simulink model "DCDC1_CL"  (R2024a)
settings: Solver=VariableStepAuto  StartTime=0.0  StopTime=Tsim_outLoop  FixedStep=Tstep  RelTol=1e-3
undefined symbols (not defined in the file): deadtimesw, den_aaf, DiscIntNeverNeededParam, ILmax, kaw_i, kaw_v, ki_i, ki_v, kp_i, kp_v, kpf_i, kpf_v, num_aaf, Rload, Tstep, Tsw, VinNom, VLlim, VoutNom, zden_pf_i, zden_pf_v, znum_pf_i, znum_pf_v
libraries: nesl_utility x12, fl_lib x11, simulink x6, ee_lib x3, spsTriangleGeneratorLib x2
settings Model: Creator=nicholas  LastModifiedBy=nicholas
settings RTWCC: GPUComputeCapability=3.5

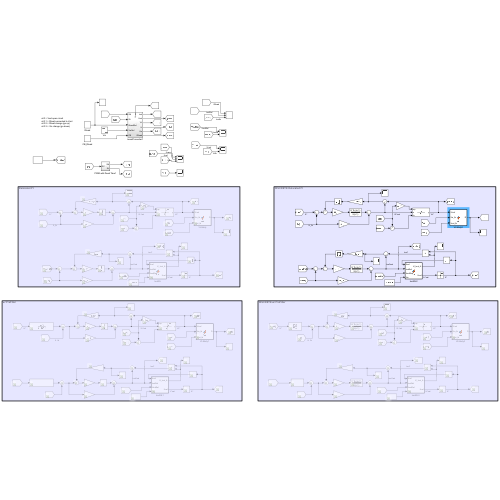
[thumbnail: Simulink's stored preview of the top-level diagram]
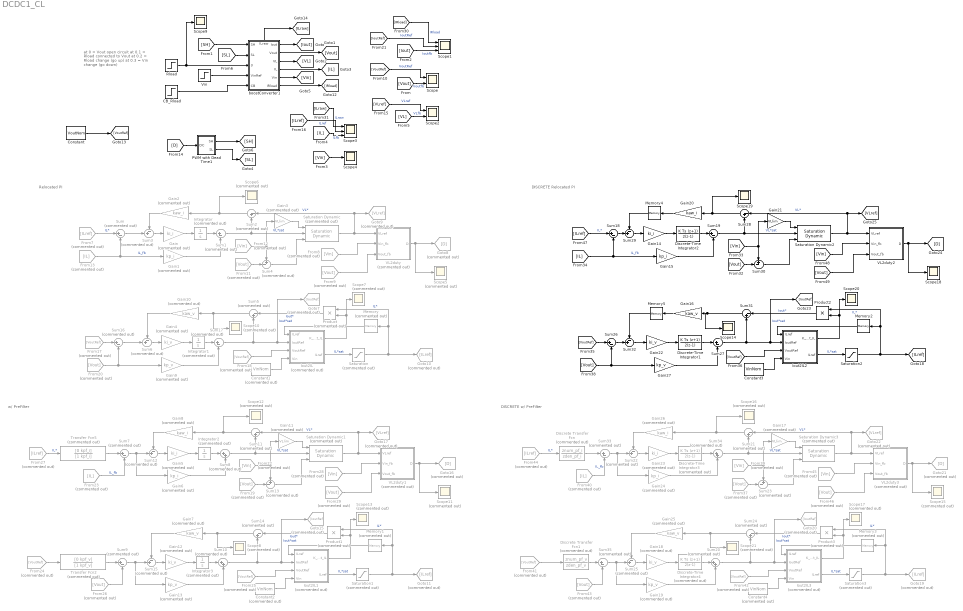
== system DCDC1_CL ==
  note: at 0 = Vout open circuit
      | at 0.1 = Rload connected to Vout
      | at 0.2 = Rload change (go up)
      | at 0.3 = Vin change (go down)
  note: Relocated PI
  note: w/ PreFilter
  note: DISCRETE w/ PreFilter
  note: DISCRETE Relocated PI
  CB_Rload : Step  Time=0.1  SampleTime=0
  Constant : Constant  Value=VoutNom
  Constant1 : Constant  Commented=on  Value=VinNom
  Constant2 : Constant  Commented=on  Value=VinNom
  Constant3 : Constant  Value=VinNom
  Constant4 : Constant  Commented=on  Value=VinNom
  Discrete Transfer Fcn : DiscreteTransferFcn  Commented=on  Numerator=znum_pf_i  Denominator=zden_pf_i
  Discrete Transfer Fcn1 : DiscreteTransferFcn  Commented=on  Numerator=znum_pf_v  Denominator=zden_pf_v
  Discrete-Time Integrator1 : DiscreteIntegrator  IntegratorMethod=Integration: Trapezoidal  SampleTime=Tsw  ICPrevOutput=DiscIntNeverNeededParam  ICPrevScaledInput=DiscIntNeverNeededParam
  Discrete-Time Integrator2 : DiscreteIntegrator  IntegratorMethod=Integration: Trapezoidal  SampleTime=Tsw  ICPrevOutput=DiscIntNeverNeededParam  ICPrevScaledInput=DiscIntNeverNeededParam
  Discrete-Time Integrator3 : DiscreteIntegrator  Commented=on  IntegratorMethod=Integration: Trapezoidal  SampleTime=Tsw  ICPrevOutput=DiscIntNeverNeededParam  ICPrevScaledInput=DiscIntNeverNeededParam
  Discrete-Time Integrator4 : DiscreteIntegrator  Commented=on  IntegratorMethod=Integration: Trapezoidal  SampleTime=Tsw  ICPrevOutput=DiscIntNeverNeededParam  ICPrevScaledInput=DiscIntNeverNeededParam
  From{9,11,19..20,26,29,37,43,46} (9 alike) : From  Commented=on  GotoTag=Vout
  From{8,12,22,28,39,45} (6 alike) : From  Commented=on  GotoTag=Vin
  From13 : From  Commented=on  GotoTag=IL
  From{17..18,24..25,41..42} (6 alike) : From  Commented=on  GotoTag=VoutRef
  From23 : From  Commented=on  GotoTag=IL
  From27 : From  Commented=on  GotoTag=ILref
  From40 : From  Commented=on  GotoTag=IL
  From44 : From  Commented=on  GotoTag=ILref
  From7 : From  Commented=on  GotoTag=ILref
  Gain : Gain  Commented=on  Gain=ki_i
  Gain1 : Gain  Commented=on  Gain=kp_i
  Gain10 : Gain  Commented=on  Gain=kaw_v
  Gain11 : Gain  Commented=on  Gain=VLlim
  Gain12 : Gain  Commented=on  Gain=ki_v
  Gain13 : Gain  Commented=on  Gain=kp_v
  Gain14 : Gain  Gain=ki_i
  Gain15 : Gain  Gain=kp_i
  Gain16 : Gain  Gain=kaw_v
  Gain17 : Gain  Commented=on  Gain=VLlim
  Gain18 : Gain  Commented=on  Gain=ki_v
  Gain19 : Gain  Commented=on  Gain=kp_v
  Gain2 : Gain  Commented=on  Gain=kaw_i
  Gain20 : Gain  Gain=kaw_i
  Gain21 : Gain  Gain=VLlim
  Gain22 : Gain  Gain=ki_v
  Gain23 : Gain  Commented=on  Gain=ki_i
  Gain24 : Gain  Commented=on  Gain=kp_i
  Gain25 : Gain  Commented=on  Gain=kaw_v
  Gain26 : Gain  Commented=on  Gain=kaw_i
  Gain27 : Gain  Gain=kp_v
  Gain3 : Gain  Commented=on  Gain=VLlim
  Gain4 : Gain  Commented=on  Gain=ki_v
  Gain5 : Gain  Commented=on  Gain=ki_i
  Gain6 : Gain  Commented=on  Gain=kp_i
  Gain7 : Gain  Commented=on  Gain=kaw_v
  Gain8 : Gain  Commented=on  Gain=kaw_i
  Gain9 : Gain  Commented=on  Gain=kp_v
  Goto10 : Goto  Commented=on  GotoTag=ILref
  Goto11 : Goto  Commented=on  GotoTag=ILref
  Goto15 : Goto  Commented=on  GotoTag=IoutRef
  Goto16 : Goto  Commented=on  GotoTag=D
  Goto17 : Goto  Commented=on  GotoTag=VLref
  Goto19 : Goto  Commented=on  GotoTag=ILref
  Goto20 : Goto  Commented=on  GotoTag=IoutRef
  Goto21 : Goto  Commented=on  GotoTag=D
  Goto22 : Goto  Commented=on  GotoTag=VLref
  Goto7 : Goto  Commented=on  GotoTag=IoutRef
  Goto8 : Goto  Commented=on  GotoTag=D
  Goto9 : Goto  Commented=on  GotoTag=VLref
  Integrator{,1..3} (4 alike) : Integrator  Commented=on
  Iout2IL : MATLAB Function  Commented=on  TreatAsAtomicUnit=on
  Iout2IL1 : MATLAB Function  Commented=on  TreatAsAtomicUnit=on
  Iout2IL2 : MATLAB Function  TreatAsAtomicUnit=on
  Iout2IL3 : MATLAB Function  Commented=on  TreatAsAtomicUnit=on
  Memory : Memory  Commented=on
  Memory1 : Memory  Commented=on
  Memory2 : Memory
  Memory3 : Memory  Commented=on
  Memory4 : Memory
  Memory5 : Memory
  PWM with Dead Time1 : Subsystem
  Product : Product  Commented=on
  Product1 : Product  Commented=on
  Product2 : Product
  Product3 : Product  Commented=on
  Rload : Step  Time=0.2  Before=Rload  After=Rload*2  SampleTime=0
  Saturation : Saturate  Commented=on  UpperLimit=ILmax  LowerLimit=-ILmax
  Saturation Dynamic : simulink/Discontinuities/Saturation Dynamic  Commented=on  OutMin=[]  OutMax=[]  OutDataTypeStr=Inherit: Same as second input  OutDataType=fixdt(1, 16)  OutScaling=2^-10  DoSatur=off
  Saturation Dynamic1 : simulink/Discontinuities/Saturation Dynamic  Commented=on  OutMin=[]  OutMax=[]  OutDataTypeStr=Inherit: Same as second input  OutDataType=fixdt(1, 16)  OutScaling=2^-10  DoSatur=off
  Saturation Dynamic2 : simulink/Discontinuities/Saturation Dynamic  OutMin=[]  OutMax=[]  OutDataTypeStr=Inherit: Same as second input  OutDataType=fixdt(1, 16)  OutScaling=2^-10  DoSatur=off
  Saturation Dynamic3 : simulink/Discontinuities/Saturation Dynamic  Commented=on  OutMin=[]  OutMax=[]  OutDataTypeStr=Inherit: Same as second input  OutDataType=fixdt(1, 16)  OutScaling=2^-10  DoSatur=off
  Saturation1 : Saturate  Commented=on  UpperLimit=ILmax  LowerLimit=-ILmax
  Saturation2 : Saturate  UpperLimit=ILmax  LowerLimit=-ILmax
  Saturation3 : Saturate  Commented=on  UpperLimit=ILmax  LowerLimit=-ILmax
  Scope : Scope  NumInputPorts=2
  Scope1 : Scope  NumInputPorts=3
  Scope{5..8,10..13,15..17,21} (12 alike) : Scope  Commented=on
  Scope{4,9,14,18..20} (6 alike) : Scope
  Scope2 : Scope  NumInputPorts=2
  Scope3 : Scope  NumInputPorts=3
  Sum{,1,7,9,16..17,33,35} (8 alike) : Sum  Commented=on  Inputs=|+-
  Sum{8,10,20,34} (4 alike) : Sum  Commented=on  Inputs=|++
  Sum{2,5,11,14,21,24} (6 alike) : Sum  Commented=on  Inputs=|-+
  Sum{3,6,12,15,22,25} (6 alike) : Sum  Commented=on  Inputs=-+|
  Sum13 : Sum  Commented=on  Inputs=+-|
  Sum{18..19,26..27} (4 alike) : Sum  Inputs=|+-
  Sum23 : Sum  Commented=on  Inputs=+-|
  Sum28 : Sum  Inputs=|-+
  Sum29 : Sum  Inputs=-+|
  Sum30 : Sum  Inputs=+-|
  Sum31 : Sum  Inputs=|-+
  Sum32 : Sum  Inputs=-+|
  Sum4 : Sum  Commented=on  Inputs=+-|
  Transfer Fcn2 : TransferFcn  Commented=on  Numerator=[0 kpf_v]  Denominator=[1 kpf_v]
  Transfer Fcn5 : TransferFcn  Commented=on  Numerator=[0 kpf_i]  Denominator=[1 kpf_i]
  VL2duty : MATLAB Function  Commented=on  TreatAsAtomicUnit=on
  VL2duty1 : MATLAB Function  Commented=on  TreatAsAtomicUnit=on
  VL2duty2 : MATLAB Function  TreatAsAtomicUnit=on
  VL2duty3 : MATLAB Function  Commented=on  TreatAsAtomicUnit=on
  Vin : Step  Time=0.3  Before=VinNom  After=20  SampleTime=0
  boostConverter1 : Subsystem
      settings: PortSchema="{\"entries\":[{\"content\":{\"sides\":[{\"content\":{\"connectorIds\":[\"In1\",\"In2\",\"In3\",\"In4\",\"In5\"]},\"type\":\"ConnectorPlacement.EquallySpacedRectSide\",\"uuid\":\"06a7732a-1944-48bb-a78f-c13d5f08aafd\"},{\"content\":{\"connectorIds\":[\"Out1\",\"Out2\",\"Out3\",\"Out4\",\"Out5\",\"Out6\"],\"side\":\"RIGHT\"},\"type\":\"ConnectorPlacement.EquallySpacedRectSide\",\"uuid\":\"b6473c2d-6993-432c-a609-70fa8f5d2a01\"},{\"content\":{\"connectorIds\":[\"Out7\"],\"side\":\"TOP\"},\"type\":\"ConnectorPlacement.EquallySpacedRectSide\",\"uuid\":\"820da1cd-7cba-427a-8731-9f11d2b16288\"}]},\"type\":\"ConnectorPlacement.EquallySpacedConnector\",\"uuid\":\"6b53f1fe-7446-41e3-8699-ec810cec24ed\"}],\"packageUris\":[\"http://schema.mathworks.com/mf0/Connector/R2020b\"],\"version\":\"1.0\"}"
  wires:
  [Vin] -> Scope4/1
  [Iout] -> Scope1/3  "Ioutfb"
  [VL] -> Scope2/2  "VLfb"
  [Vout] -> Scope/2  "Voutfb"
  [IL] -> Scope3/3  "ILfb"
  boostConverter1/1(Iout) -> [Iout]
  boostConverter1/2(Vout) -> [Vout]
  boostConverter1/3(VL) -> [VL]
  boostConverter1/4(IL) -> [IL]
  boostConverter1/5(Vin) -> [Vin]
  [SL] -> boostConverter1/2(SL)
  [SH] -> boostConverter1/1(SH)
  [D] -> PWM with Dead Time1/1(DC)
  PWM with Dead Time1/1(SH) -> [SH]
  PWM with Dead Time1/2(SL) -> [SL]
  [VLref] -> Scope2/1  "VLref"
  [ILref] -> Scope3/2  "ILref"
  Rload/1 -> boostConverter1/3(RloadRef), Scope9/1
  [VoutRef] -> Scope/1  "VoutRef"
  [IoutRef] -> Scope1/2  "IoutRef"
  Constant/1 -> [VoutRef]
  From11/1 -> Sum4/2
  Gain3/1 -> Saturation Dynamic/1
  Saturation Dynamic/1 -> VL2duty/1(VLref), Sum2/1, Goto9/1  "VL*"
  Sum4/1 -> Saturation Dynamic/3
  Integrator/1 -> Sum1/1
  Gain1/1 -> Sum1/2
  Sum/1 -> Sum3/2
  Sum3/1 -> Gain/1
  VL2duty/1(D) -> Scope5/1, Goto8/1
  Sum2/1 -> Scope6/1, Gain2/1
  From13/1 -> Gain1/1, Sum/2  "IL_fb"
  From12/1 -> Gain3/1, Sum4/1
  Sum1/1 -> Saturation Dynamic/2, Sum2/2  "VL*sat"
  From7/1 -> Sum/1  "IL*"
  From8/1 -> VL2duty/2(Vin_fb)
  Gain/1 -> Integrator/1
  From9/1 -> VL2duty/3(Vout_fb)
  Gain2/1 -> Sum3/1
  Saturation/1 -> Product/1, Memory/1, Goto10/1  "IL*"
  Constant1/1 -> Iout2IL/4(Vin)
  Product/1 -> Sum5/1  "Iout*"
  Gain10/1 -> Sum6/1
  Iout2IL/2(ILref) -> Saturation/1  "IL*sat"
  Gain4/1 -> Integrator1/1
  Iout2IL/1(K_Iout_IL) -> Product/2, Scope7/1
  Sum6/1 -> Gain4/1
  Sum5/1 -> Scope10/1, Gain10/1
  Gain9/1 -> Sum17/2
  Sum16/1 -> Sum6/2
  Sum17/1 -> Sum5/2, Goto7/1, Iout2IL/2(IoutRef)  "Iout*sat"
  From17/1 -> Sum16/1
  Memory/1 -> Iout2IL/1("ILref ")
  From18/1 -> Iout2IL/3(VoutRef)
  Integrator1/1 -> Sum17/1
  From20/1 -> Gain9/1, Sum16/2
  From19/1 -> Sum13/2
  Gain11/1 -> Saturation Dynamic1/1
  From22/1 -> Gain11/1, Sum13/1
  Sum7/1 -> Gain6/1, Sum12/2
  Saturation Dynamic1/1 -> VL2duty1/1(VLref), Sum11/1, Goto17/1  "VL*"
  Sum8/1 -> Saturation Dynamic1/2, Sum11/2  "VL*sat"
  From23/1 -> Sum7/2  "IL_fb"
  Sum12/1 -> Gain5/1
  Integrator2/1 -> Sum8/1
  Sum13/1 -> Saturation Dynamic1/3
  From26/1 -> Sum9/2
  Integrator3/1 -> Sum10/1
  Gain6/1 -> Sum8/2
  Iout2IL1/2(ILref) -> Saturation1/1  "IL*sat"
  Saturation1/1 -> Product1/1, Memory1/1, Goto11/1  "IL*"
  From24/1 -> Transfer Fcn2/1
  Sum10/1 -> Sum14/2, Iout2IL1/2(IoutRef), Goto15/1  "Iout*sat"
  Gain5/1 -> Integrator2/1
  Gain12/1 -> Integrator3/1
  Sum14/1 -> Scope8/1, Gain7/1
  Gain8/1 -> Sum12/1
  Memory1/1 -> Iout2IL1/1("ILref ")
  Sum15/1 -> Gain12/1
  Gain7/1 -> Sum15/1
  Gain13/1 -> Sum10/2
  Sum11/1 -> Scope12/1, Gain8/1
  Sum9/1 -> Gain13/1, Sum15/2
  Product1/1 -> Sum14/1  "Iout*"
  Iout2IL1/1(K_Iout_IL) -> Product1/2, Scope13/1
  Constant2/1 -> Iout2IL1/4(Vin)
  From25/1 -> Iout2IL1/3(VoutRef)
  From27/1 -> Transfer Fcn5/1  "IL*"
  From29/1 -> VL2duty1/3(Vout_fb)
  From28/1 -> VL2duty1/2(Vin_fb)
  VL2duty1/1(D) -> Scope11/1, Goto16/1
  Transfer Fcn2/1 -> Sum9/1
  Transfer Fcn5/1 -> Sum7/1
  Vin/1 -> boostConverter1/4(VinRef)
  CB_Rload/1 -> boostConverter1/5(CB)
  boostConverter1/6(IRload) -> [IRload]
  [IRload] -> Scope1/1  "IRload"
  boostConverter1/7(ILraw) -> [ILraw]
  [ILraw] -> Scope3/1  "ILraw"
  VL2duty3/1(D) -> Scope15/1, Goto21/1
  From41/1 -> Discrete Transfer Fcn1/1
  VL2duty2/1(D) -> Scope18/1, [D]
  From44/1 -> Discrete Transfer Fcn/1  "IL*"
  Gain14/1 -> Discrete-Time Integrator2/1
  Sum24/1 -> Scope21/1, Gain25/1
  Discrete Transfer Fcn/1 -> Sum33/1
  Discrete Transfer Fcn1/1 -> Sum35/1
  Sum20/1 -> Sum24/2, Iout2IL3/2(IoutRef), Goto20/1  "Iout*sat"
  Gain26/1 -> Sum22/1
  Gain17/1 -> Saturation Dynamic3/1
  Sum30/1 -> Saturation Dynamic2/3
  Gain25/1 -> Sum25/1
  From42/1 -> Iout2IL3/3(VoutRef)
  From37/1 -> Sum23/2
  From40/1 -> Sum33/2  "IL_fb"
  Gain23/1 -> Discrete-Time Integrator3/1
  Iout2IL3/2(ILref) -> Saturation3/1  "IL*sat"
  [VoutRef] -> Sum26/1
  [IL] -> Gain15/1, Sum18/2  "IL_fb"
  From45/1 -> VL2duty3/2(Vin_fb)
  From46/1 -> VL2duty3/3(Vout_fb)
  Iout2IL2/2(ILref) -> Saturation2/1  "IL*sat"
  Constant4/1 -> Iout2IL3/4(Vin)
  Saturation3/1 -> Product3/1, Memory3/1, Goto19/1  "IL*"
  [Vin] -> VL2duty2/2(Vin_fb)
  Sum19/1 -> Saturation Dynamic2/2, Sum28/2  "VL*sat"
  Sum21/1 -> Scope16/1, Gain26/1
  Gain19/1 -> Sum20/2
  Sum35/1 -> Gain19/1, Sum25/2
  Product3/1 -> Sum24/1  "Iout*"
  Discrete-Time Integrator4/1 -> Sum20/1
  Sum25/1 -> Gain18/1
  Sum18/1 -> Sum29/2
  Gain21/1 -> Saturation Dynamic2/1
  [ILref] -> Sum18/1  "IL*"
  Gain24/1 -> Sum34/2
  Sum31/1 -> Scope14/1, Gain16/1
  Product2/1 -> Sum31/1  "Iout*"
  From39/1 -> Gain17/1, Sum23/1
  Memory3/1 -> Iout2IL3/1("ILref ")
  Discrete-Time Integrator3/1 -> Sum34/1
  Sum23/1 -> Saturation Dynamic3/3
  Memory2/1 -> Iout2IL2/1("ILref ")
  Sum22/1 -> Gain23/1
  Sum34/1 -> Saturation Dynamic3/2, Sum21/2  "VL*sat"
  [Vout] -> Sum30/2
  Iout2IL3/1(K_Iout_IL) -> Product3/2, Scope17/1
  [VoutRef] -> Iout2IL2/3(VoutRef)
  Gain16/1 -> Memory5/1
  Gain18/1 -> Discrete-Time Integrator4/1
  Discrete-Time Integrator1/1 -> Sum27/1
  Gain27/1 -> Sum27/2
  Gain15/1 -> Sum19/2
  [Vout] -> Gain27/1, Sum26/2
  Saturation Dynamic3/1 -> VL2duty3/1(VLref), Sum21/1, Goto22/1  "VL*"
  Sum26/1 -> Sum32/2
  Sum33/1 -> Gain24/1, Sum22/2
  Iout2IL2/1(K_Iout_IL) -> Product2/2, Scope20/1
  [Vout] -> VL2duty2/3(Vout_fb)
  Sum32/1 -> Gain22/1
  Discrete-Time Integrator2/1 -> Sum19/1
  Sum28/1 -> Scope19/1, Gain20/1
  Gain20/1 -> Memory4/1
  Sum27/1 -> Sum31/2, [IoutRef], Iout2IL2/2(IoutRef)  "Iout*sat"
  [Vin] -> Gain21/1, Sum30/1
  From43/1 -> Sum35/2
  Saturation2/1 -> Product2/1, Memory2/1, [ILref]  "IL*"
  Saturation Dynamic2/1 -> Sum28/1, [VLref], VL2duty2/1(VLref)  "VL*"
  Sum29/1 -> Gain14/1
  Constant3/1 -> Iout2IL2/4(Vin)
  Gain22/1 -> Discrete-Time Integrator1/1
  Memory4/1 -> Sum29/1
  Memory5/1 -> Sum32/1

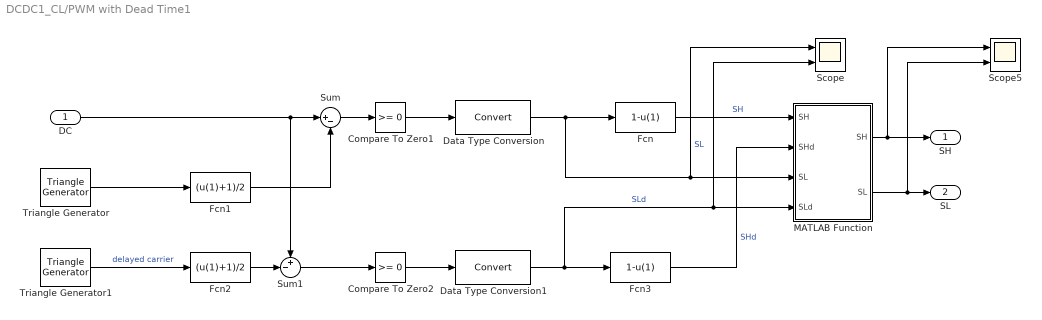
== system DCDC1_CL/PWM with Dead Time1 ==
  DC : Inport
  Compare To Zero1 : simulink/Logic and Bit Operations/Compare To Zero  relop=>=  OutDataTypeStr=boolean
  Compare To Zero2 : simulink/Logic and Bit Operations/Compare To Zero  relop=>=  OutDataTypeStr=boolean
  Data Type Conversion : DataTypeConversion  SaturateOnIntegerOverflow=off  RndMeth=Floor
  Data Type Conversion1 : DataTypeConversion  SaturateOnIntegerOverflow=off  RndMeth=Floor
  Fcn : Fcn  Expr=1-u(1)
  Fcn1 : Fcn  Expr=(u(1)+1)/2
  Fcn2 : Fcn  Expr=(u(1)+1)/2
  Fcn3 : Fcn  Expr=1-u(1)
  MATLAB Function : MATLAB Function  TreatAsAtomicUnit=on
  Scope : Scope  NumInputPorts=2
  Scope5 : Scope  NumInputPorts=2
  Sum : Sum  Inputs=|+-
  Sum1 : Sum  Inputs=+-|
  Triangle Generator : spsTriangleGeneratorLib/Triangle Generator  Freq=fsw  Phase=0  Ts=Tstep
  Triangle Generator1 : spsTriangleGeneratorLib/Triangle Generator  Freq=fsw  Phase=-(deadtimesw/Tsw)*360  Ts=Tstep
  SH : Outport
  SL : Outport  Port=2
  wires:
  Data Type Conversion/1 -> Fcn/1, Scope/1, MATLAB Function/3("SL ")  "SL"
  Fcn/1 -> MATLAB Function/1("SH ")  "SH"
  MATLAB Function/2(SL) -> SL/1, Scope5/2
  MATLAB Function/1(SH) -> SH/1, Scope5/1
  DC/1 -> Sum1/1, Sum/1
  Triangle Generator/1 -> Fcn1/1
  Sum/1 -> Compare To Zero1/1
  Fcn1/1 -> Sum/2
  Compare To Zero1/1 -> Data Type Conversion/1
  Triangle Generator1/1 -> Fcn2/1  "delayed carrier"
  Sum1/1 -> Compare To Zero2/1
  Compare To Zero2/1 -> Data Type Conversion1/1
  Fcn2/1 -> Sum1/2
  Data Type Conversion1/1 -> Fcn3/1, Scope/2, MATLAB Function/4(SLd)  "SLd"
  Fcn3/1 -> MATLAB Function/2(SHd)  "SHd"

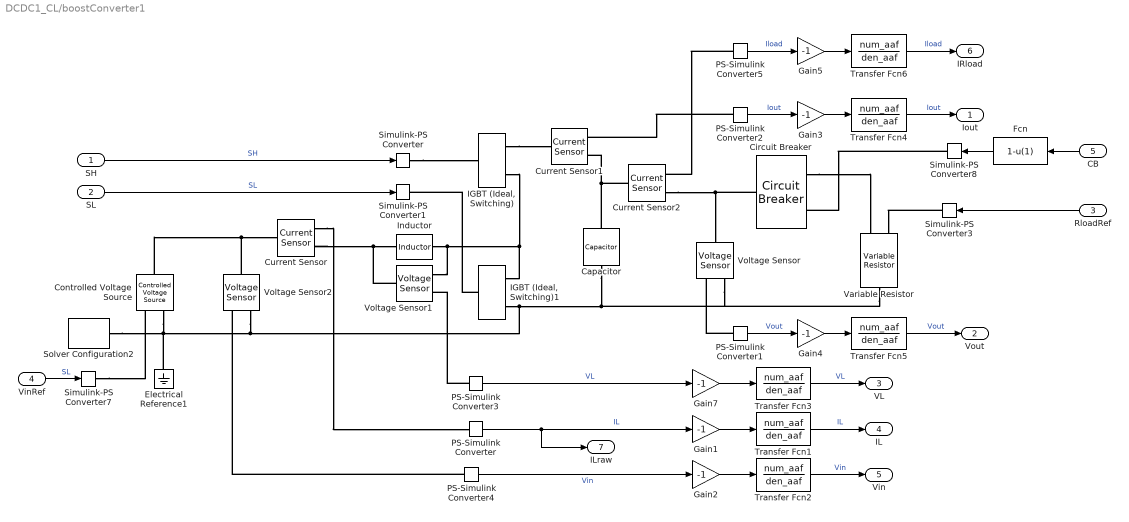
== system DCDC1_CL/boostConverter1 ==
  SH : Inport
  SL : Inport  Port=2
  RloadRef : Inport  Port=3
  VinRef : Inport  Port=4
  CB : Inport  Port=5
  Capacitor : fl_lib/Electrical/Electrical Elements/Capacitor  c=C F  r=ResrC Ohm  g=0 1/Ohm  i_specify=off  i_priority=None  i=0 A  i_nominal_specify=off  i_nominal_value=1  i_nominal_unit=A  v_specify=off  v_priority=High  v=VoutNom V  v_nominal_specify=off  v_nominal_value=1  v_nominal_unit=V  vc_specify=off  vc_priority=High  vc=0 V  vc_nominal_specify=off  vc_nominal_value=1  vc_nominal_unit=V
  Circuit Breaker : ee_lib/Switches & Breakers/Circuit Breaker  R_closed=0.001 Ohm  G_open=1e-12 1/Ohm  threshold=0.5 V  breaker_behavior=ee.enum.switches.breakerBehavior.zeroCrossingDisable
      settings: InternalSimscapePortConfiguration="{\"Bottom\":[],\"Left\":[{\"id\":\"vT\",\"label\":\"vT\",\"type\":\"input\"},{\"id\":\"p1\",\"label\":\"\",\"type\":\"foundation.electrical.electrical\"}],\"Right\":[{\"id\":\"p2\",\"label\":\"\",\"type\":\"foundation.electrical.electrical\"}],\"Top\":[]}"
  Controlled Voltage Source : fl_lib/Electrical/Electrical Sources/Controlled Voltage Source
  Current Sensor : fl_lib/Electrical/Electrical Sensors/Current Sensor
  Current Sensor1 : fl_lib/Electrical/Electrical Sensors/Current Sensor
  Current Sensor2 : fl_lib/Electrical/Electrical Sensors/Current Sensor
  Electrical Reference1 : fl_lib/Electrical/Electrical Elements/Electrical Reference
  Fcn : Fcn  Expr=1-u(1)
  Gain{1..5,7} (6 alike) : Gain  Gain=-1
  "IGBT (Ideal, Switching)" : ee_lib/Semiconductors & Converters/IGBT (Ideal, Switching)  port_option=ee.enum.controlport.ps  Vf=0.8 V  Ron=0.001 Ohm  Goff=1e-5 1/Ohm  Vth=VthIGBT V  diode_param=ee.enum.converters.protectiondiode.nodynamics  diode_Vf=0.8 V  diode_Ron=0.001 Ohm  diode_Goff=1e-5 1/Ohm  diode_C=50e-9 F  diode_iRM=-235 A  diode_iF=300 A  diode_idot=-50 A/us  diode_trr_param=ee.enum.converters.diodeReverseParam.trr_factor  diode_trr_factor=3  diode_trr=15 us  diode_Qrr=1500 s*uA  ice_specify=off  ice_priority=None  ice=0 A  ice_nominal_specify=off  ice_nominal_value=1  ice_nominal_unit=A  vce_specify=off  vce_priority=None  vce=0 V  vce_nominal_specify=off  vce_nominal_value=1  vce_nominal_unit=V  vge_specify=off  vge_priority=None  vge=0 V  vge_nominal_specify=off  vge_nominal_value=1  vge_nominal_unit=V  thermal_loss_option=ee.enum.converters.thermalLossOption.constantvalues  Von_data=[0, .1, .6, .8, 1, 1.3, 1.6, 2, 2.4; 0, .1, .7, 1, 1.2, 1.5, 1.9, 2.4, 2.8] V  Tj=[298.15, 398.15] K  Iout_data=[0, .1, 1, 5, 10, 20, 40, 70, 100] A  Eon_data=[0, .0024, .024, .12, .2, .48, 1.04, 2.16, 3.24; 0, .003, .03, .15, .25, .6, 1.3, 2.7, 4.05] * 1e-3 J  Eoff_data=[0, .0007, .0066, .033, .066, .17, .33, .83, 1.5; 0, .001, .01, .05, .1, .25, .5, 1.2, 2.2] * 1e-3 J  Eon_data_3D=[zeros(2, 9, 3)] J  Eoff_data_3D=[zeros(2, 9, 3)] J  Tj_loss=[298.15, 398.15] K  Iout_data_loss=[0, .1, 1, 5, 10, 20, 40, 70, 100] A  tabulateWithVce=false  Vce_loss=[0, 150, 300] V  Eon_scalar=22.86e-3 J  Eoff_scalar=17.14e-3 J  Voff=300 V  Iout_scalar=600 A  useCurrentFromPreviousCycle=false  useVoltageFromPreviousCycle=false  diodeModelType=ee.enum.converters.diodeModelType.pwl  diodeTableType=ee.enum.diode.tableType.IfMat  diode_ReverseIVType=ee.enum.diode.diodeReverseIV.constant  diode_IfMat=[.07, .12, .19, 1.75, 4.24, 7.32, 11.2; .16, .3, .72, 2.14, 4.02, 6.35, 9.12] A  diode_VfMat=[.9, 1.15, 1.25, 1.5, 1.75, 2.17, 2.6, 2.85; .58, .68, .75, 1.1, 1.38, 1.77, 2.27, 2.7] V  diode_TjVec=[25, 125] degC  diode_VfVec=[.5, .7, .9, 1.3, 1.7, 2.1, 2.5] V  diode_IfVec=[.1, .2, .5, 1, 2, 4, 7, 10] A  diode_IrMat=[1e-06, 2e-06, 5e-06, 1e-05, 2.5e-05, 5e-05, .0001; 2e-06, 5e-06, 1e-05, 4e-05, 8e-05, .0002, .0005] A  diode_VrMat=[10, 100, 200, 250, 300, 325, 350; 10, 70, 160, 220, 270, 300, 320] V  diode_VrVec=[10, 20, 40, 50, 70, 80, 100] V  diode_IrVec=[1e-06, 2e-06, 5e-06, 1e-05, 2e-05, 5e-05, .0001] A  diode_Vr=-600 V  diode_Ls=150 nH  diode_Erec=0.03 J  diode_rec_loss_model=ee.enum.diode.reverseRecoveryModel.fixed  diode_ErecVal=0 J  diode_scaleWithIandV=true  diode_ErecMat=zeros(2, 3) J  diode_TjrecVec=[298.15, 398.15] K  diode_IfrecVec=[.1, 1, 10] A  diode_IrecVal=10 A  diode_VrecVal=10 V  diode_tFilter=1 / 1000 / 100 s  thermal_network_parameterization=ee.enum.thermalNetworkTopology.external  Rth=[.08, .5] K/W  Rth_Cauer=[.08, .1, .5] K/W  Rth_Foster=[.08, .14, .22, .16] K/W  thermal_mass_parameterization=ee.enum.thermalNetwork.timeconstant  thermal_mass=[.01, .5] J/K  thermal_mass_Cauer=[.01, .1, .5] J/K  thermal_mass_Foster=[.001, .005, .05, .5] J/K  thermal_time_constant=[.001, .2] s  thermal_time_constant_Cauer=[.001, .1, .2] s  thermal_time_constant_Foster=[7e-05, .0007, .01, .08] s  thermal_mass_initial_temperatures=[25, 25] degC  thermal_mass_initial_temperatures_Cauer=[25, 25, 25] degC  junction_thermal_mass=0.01 J/K  Tvec_initial_Foster=[25, 25, 25, 25] degC  no_thermal_network=0  junction_temperature_specify=off  junction_temperature_priority=None  junction_temperature=25 degC  junction_temperature_nominal_specify=off  junction_temperature_nominal_value=1  junction_temperature_nominal_unit=degC  Qj_specify=off  Qj_priority=None  Qj=0 W  Qj_nominal_specify=off  Qj_nominal_value=1  Qj_nominal_unit=W  accumulatedSwitchingLosses_specify=off  accumulatedSwitchingLosses_priority=None  accumulatedSwitchingLosses=0 J
  "IGBT (Ideal, Switching)1" : ee_lib/Semiconductors & Converters/IGBT (Ideal, Switching)  port_option=ee.enum.controlport.ps  Vf=0.8 V  Ron=0.001 Ohm  Goff=1e-5 1/Ohm  Vth=VthIGBT V  diode_param=ee.enum.converters.protectiondiode.nodynamics  diode_Vf=0.8 V  diode_Ron=0.001 Ohm  diode_Goff=1e-5 1/Ohm  diode_C=50e-9 F  diode_iRM=-235 A  diode_iF=300 A  diode_idot=-50 A/us  diode_trr_param=ee.enum.converters.diodeReverseParam.trr_factor  diode_trr_factor=3  diode_trr=15 us  diode_Qrr=1500 s*uA  ice_specify=off  ice_priority=None  ice=0 A  ice_nominal_specify=off  ice_nominal_value=1  ice_nominal_unit=A  vce_specify=off  vce_priority=None  vce=0 V  vce_nominal_specify=off  vce_nominal_value=1  vce_nominal_unit=V  vge_specify=off  vge_priority=None  vge=0 V  vge_nominal_specify=off  vge_nominal_value=1  vge_nominal_unit=V  thermal_loss_option=ee.enum.converters.thermalLossOption.constantvalues  Von_data=[0, .1, .6, .8, 1, 1.3, 1.6, 2, 2.4; 0, .1, .7, 1, 1.2, 1.5, 1.9, 2.4, 2.8] V  Tj=[298.15, 398.15] K  Iout_data=[0, .1, 1, 5, 10, 20, 40, 70, 100] A  Eon_data=[0, .0024, .024, .12, .2, .48, 1.04, 2.16, 3.24; 0, .003, .03, .15, .25, .6, 1.3, 2.7, 4.05] * 1e-3 J  Eoff_data=[0, .0007, .0066, .033, .066, .17, .33, .83, 1.5; 0, .001, .01, .05, .1, .25, .5, 1.2, 2.2] * 1e-3 J  Eon_data_3D=[zeros(2, 9, 3)] J  Eoff_data_3D=[zeros(2, 9, 3)] J  Tj_loss=[298.15, 398.15] K  Iout_data_loss=[0, .1, 1, 5, 10, 20, 40, 70, 100] A  tabulateWithVce=false  Vce_loss=[0, 150, 300] V  Eon_scalar=22.86e-3 J  Eoff_scalar=17.14e-3 J  Voff=300 V  Iout_scalar=600 A  useCurrentFromPreviousCycle=false  useVoltageFromPreviousCycle=false  diodeModelType=ee.enum.converters.diodeModelType.pwl  diodeTableType=ee.enum.diode.tableType.IfMat  diode_ReverseIVType=ee.enum.diode.diodeReverseIV.constant  diode_IfMat=[.07, .12, .19, 1.75, 4.24, 7.32, 11.2; .16, .3, .72, 2.14, 4.02, 6.35, 9.12] A  diode_VfMat=[.9, 1.15, 1.25, 1.5, 1.75, 2.17, 2.6, 2.85; .58, .68, .75, 1.1, 1.38, 1.77, 2.27, 2.7] V  diode_TjVec=[25, 125] degC  diode_VfVec=[.5, .7, .9, 1.3, 1.7, 2.1, 2.5] V  diode_IfVec=[.1, .2, .5, 1, 2, 4, 7, 10] A  diode_IrMat=[1e-06, 2e-06, 5e-06, 1e-05, 2.5e-05, 5e-05, .0001; 2e-06, 5e-06, 1e-05, 4e-05, 8e-05, .0002, .0005] A  diode_VrMat=[10, 100, 200, 250, 300, 325, 350; 10, 70, 160, 220, 270, 300, 320] V  diode_VrVec=[10, 20, 40, 50, 70, 80, 100] V  diode_IrVec=[1e-06, 2e-06, 5e-06, 1e-05, 2e-05, 5e-05, .0001] A  diode_Vr=-600 V  diode_Ls=150 nH  diode_Erec=0.03 J  diode_rec_loss_model=ee.enum.diode.reverseRecoveryModel.fixed  diode_ErecVal=0 J  diode_scaleWithIandV=true  diode_ErecMat=zeros(2, 3) J  diode_TjrecVec=[298.15, 398.15] K  diode_IfrecVec=[.1, 1, 10] A  diode_IrecVal=10 A  diode_VrecVal=10 V  diode_tFilter=1 / 1000 / 100 s  thermal_network_parameterization=ee.enum.thermalNetworkTopology.external  Rth=[.08, .5] K/W  Rth_Cauer=[.08, .1, .5] K/W  Rth_Foster=[.08, .14, .22, .16] K/W  thermal_mass_parameterization=ee.enum.thermalNetwork.timeconstant  thermal_mass=[.01, .5] J/K  thermal_mass_Cauer=[.01, .1, .5] J/K  thermal_mass_Foster=[.001, .005, .05, .5] J/K  thermal_time_constant=[.001, .2] s  thermal_time_constant_Cauer=[.001, .1, .2] s  thermal_time_constant_Foster=[7e-05, .0007, .01, .08] s  thermal_mass_initial_temperatures=[25, 25] degC  thermal_mass_initial_temperatures_Cauer=[25, 25, 25] degC  junction_thermal_mass=0.01 J/K  Tvec_initial_Foster=[25, 25, 25, 25] degC  no_thermal_network=0  junction_temperature_specify=off  junction_temperature_priority=None  junction_temperature=25 degC  junction_temperature_nominal_specify=off  junction_temperature_nominal_value=1  junction_temperature_nominal_unit=degC  Qj_specify=off  Qj_priority=None  Qj=0 W  Qj_nominal_specify=off  Qj_nominal_value=1  Qj_nominal_unit=W  accumulatedSwitchingLosses_specify=off  accumulatedSwitchingLosses_priority=None  accumulatedSwitchingLosses=0 J
  Inductor : fl_lib/Electrical/Electrical Elements/Inductor  l=L H  r=RserL Ohm  g=1e-9 1/Ohm  i_specify=off  i_priority=None  i=Iin A  i_nominal_specify=off  i_nominal_value=1  i_nominal_unit=A  v_specify=off  v_priority=None  v=0 V  v_nominal_specify=off  v_nominal_value=1  v_nominal_unit=V  i_L_specify=off  i_L_priority=High  i_L=0 A  i_L_nominal_specify=off  i_L_nominal_value=1  i_L_nominal_unit=A
  PS-Simulink Converter{,1..5} (6 alike) : nesl_utility/PS-Simulink Converter  PhysicalDomain=network_engine_domain  SubClassName=ps_output  LeftPortType=input  RightPortType=output  PseudoPeriodic=off  Frequencies=[]  VectorFormat=inherit  Unit=inherit  AffineConversion=off
  Simulink-PS Converter : nesl_utility/Simulink-PS Converter  PhysicalDomain=network_engine_domain  SubClassName=ps_input  LeftPortType=input  RightPortType=output  PseudoPeriodic=off  Frequencies=[]  NoiseDistribution=none  NoiseParameters=[]  Unit=1  AffineConversion=off  FilteringAndDerivatives=provide  SimscapeFilterOrder=1  InputFilterTimeConstant=0.001  UdotUserProvided=0
  Simulink-PS Converter1 : nesl_utility/Simulink-PS Converter  PhysicalDomain=network_engine_domain  SubClassName=ps_input  LeftPortType=input  RightPortType=output  PseudoPeriodic=off  Frequencies=[]  NoiseDistribution=none  NoiseParameters=[]  Unit=1  AffineConversion=off  FilteringAndDerivatives=provide  SimscapeFilterOrder=1  InputFilterTimeConstant=0.001  UdotUserProvided=0
  Simulink-PS Converter3 : nesl_utility/Simulink-PS Converter  PhysicalDomain=network_engine_domain  SubClassName=ps_input  LeftPortType=input  RightPortType=output  PseudoPeriodic=off  Frequencies=[]  NoiseDistribution=none  NoiseParameters=[]  Unit=1  AffineConversion=off  FilteringAndDerivatives=filter  SimscapeFilterOrder=1  InputFilterTimeConstant=Tstep  UdotUserProvided=0
  Simulink-PS Converter7 : nesl_utility/Simulink-PS Converter  PhysicalDomain=network_engine_domain  SubClassName=ps_input  LeftPortType=input  RightPortType=output  PseudoPeriodic=off  Frequencies=[]  NoiseDistribution=none  NoiseParameters=[]  Unit=1  AffineConversion=off  FilteringAndDerivatives=filter  SimscapeFilterOrder=1  InputFilterTimeConstant=Tstep  UdotUserProvided=0
  Simulink-PS Converter8 : nesl_utility/Simulink-PS Converter  PhysicalDomain=network_engine_domain  SubClassName=ps_input  LeftPortType=input  RightPortType=output  PseudoPeriodic=off  Frequencies=[]  NoiseDistribution=none  NoiseParameters=[]  Unit=1  AffineConversion=off  FilteringAndDerivatives=provide  SimscapeFilterOrder=1  InputFilterTimeConstant=0.001  UdotUserProvided=0
  Solver Configuration2 : nesl_utility/Solver Configuration  PhysicalDomain=network_engine_domain  SubClassName=solver  LeftPortType=input  RightPortType=generic  Tones=[]  Harmonics=[]  SimulateNoise=off  Profile=off  UseLocalSampling=off  EnableSwitchedLinearOptims=on  FrequencyDomain=off  UseCCode=off  RelTol=0.001  AbsTol=1e-06  MinStep=1e-09  ToWorkspace=off  RevertToSquareIcSolve=off  NumHomotopyIterations=100  PhasorMode=off  PhasorModeNumHarmonics=1  ConsistencySolver=NEWTON_FTOL  IndexReductionMethod=DerivativeReplacement  DoDC=off  ResidualTolerance=1e-09  ConsistencyTolSource=GLOBAL  ConsistencyAbsTol=0.001  ConsistencyRelTol=0.001  ConsistencyTolFactor=0.001  UseLocalSolver=off  LocalSolverChoice=NE_TRAPEZOIDAL_ADVANCER  ResolveIndetEquations=on  FunctionEvalNumThread=1  LocalSolverSampleTime=Tstep  DoFixedCost=off  MaxNonlinIter=3  MaxModeIter=2  ComputeImpulses=off  ImpulseIterations=2  LinearAlgebra=auto  LinearAlgebraNumThread=0  EquationFormulation=NE_TIME_EF  DelaysMemoryBudget=1024  AutomaticFiltering=off  FilteringTimeConstant=0.001  PartitionStorageMethod=AS_NEEDED  PartitionMemoryBudget=1024  PartitionMethod=ROBUST  MultibodyUseLocalSolver=off  MultibodyLocalSolverChoice=ODE1  MultibodyLocalSolverSampleTime=0.001
  Transfer Fcn{1..6} (6 alike) : TransferFcn  Numerator=num_aaf  Denominator=den_aaf
  Variable Resistor : fl_lib/Electrical/Electrical Elements/Variable Resistor  Rmin=Rload*0.9 Ohm  thermalEnable=false  thermal_mass=1 J/K  i_specify=off  i_priority=None  i=0 A  i_nominal_specify=off  i_nominal_value=1  i_nominal_unit=A  v_specify=off  v_priority=None  v=0 V  v_nominal_specify=off  v_nominal_value=1  v_nominal_unit=V  T_specify=off  T_priority=None  T=300 K  T_nominal_specify=off  T_nominal_value=1  T_nominal_unit=K
  Voltage Sensor : fl_lib/Electrical/Electrical Sensors/Voltage Sensor
  Voltage Sensor1 : fl_lib/Electrical/Electrical Sensors/Voltage Sensor
  Voltage Sensor2 : fl_lib/Electrical/Electrical Sensors/Voltage Sensor
  Iout : Outport
  Vout : Outport  Port=2
  VL : Outport  Port=3
  IL : Outport  Port=4
  Vin : Outport  Port=5
  IRload : Outport  Port=6
  ILraw : Outport  Port=7
  wires:
  PS-Simulink Converter4/1 -> Gain2/1  "Vin"
  SH/1 -> Simulink-PS Converter/1  "SH"
  PS-Simulink Converter2/1 -> Gain3/1  "Iout"
  PS-Simulink Converter1/1 -> Gain4/1  "Vout"
  PS-Simulink Converter/1 -> ILraw/1, Gain1/1  "IL"
  PS-Simulink Converter3/1 -> Gain7/1  "VL"
  SL/1 -> Simulink-PS Converter1/1  "SL"
  Transfer Fcn3/1 -> VL/1  "VL"
  Gain7/1 -> Transfer Fcn3/1
  Transfer Fcn1/1 -> IL/1  "IL"
  Transfer Fcn2/1 -> Vin/1  "Vin"
  Transfer Fcn4/1 -> Iout/1  "Iout"
  Gain1/1 -> Transfer Fcn1/1
  Gain2/1 -> Transfer Fcn2/1
  Gain3/1 -> Transfer Fcn4/1
  RloadRef/1 -> Simulink-PS Converter3/1
  Transfer Fcn5/1 -> Vout/1  "Vout"
  Gain4/1 -> Transfer Fcn5/1
  Gain5/1 -> Transfer Fcn6/1
  Transfer Fcn6/1 -> IRload/1  "Iload"
  VinRef/1 -> Simulink-PS Converter7/1  "SL"
  CB/1 -> Fcn/1
  PS-Simulink Converter5/1 -> Gain5/1  "Iload"
  Fcn/1 -> Simulink-PS Converter8/1
  connections:
  Current Sensor/RConn1 -- PS-Simulink Converter/LConn1
  Current Sensor/RConn2 -- Voltage Sensor1/LConn1 -- Inductor/LConn1
  Solver Configuration2/RConn1 -- Electrical Reference1/LConn1 -- "IGBT (Ideal, Switching)1"/RConn2 -- Capacitor/RConn1 -- Variable Resistor/RConn1 -- Voltage Sensor/RConn2 -- Voltage Sensor2/RConn2 -- Controlled Voltage Source/RConn2
  PS-Simulink Converter4/LConn1 -- Voltage Sensor2/RConn1
  Voltage Sensor2/LConn1 -- Current Sensor/LConn1 -- Controlled Voltage Source/LConn1
  Current Sensor2/RConn2 -- Voltage Sensor/LConn1 -- Circuit Breaker/RConn1
  Inductor/RConn1 -- Voltage Sensor1/RConn2 -- "IGBT (Ideal, Switching)1"/RConn1 -- "IGBT (Ideal, Switching)"/RConn2
  PS-Simulink Converter3/LConn1 -- Voltage Sensor1/RConn1
  "IGBT (Ideal, Switching)"/RConn1 -- Current Sensor1/LConn1
  "IGBT (Ideal, Switching)1"/LConn1 -- Simulink-PS Converter1/RConn1
  PS-Simulink Converter2/LConn1 -- Current Sensor1/RConn1
  PS-Simulink Converter1/LConn1 -- Voltage Sensor/RConn1
  Simulink-PS Converter/RConn1 -- "IGBT (Ideal, Switching)"/LConn1
  Simulink-PS Converter7/RConn1 -- Controlled Voltage Source/RConn1
  Simulink-PS Converter8/RConn1 -- Circuit Breaker/LConn1
  Current Sensor2/LConn1 -- Capacitor/LConn1 -- Current Sensor1/RConn2
  Circuit Breaker/LConn2 -- Variable Resistor/LConn2
  Simulink-PS Converter3/RConn1 -- Variable Resistor/LConn1
  PS-Simulink Converter5/LConn1 -- Current Sensor2/RConn1

== matlab function DCDC1_CL/VL2duty3 ==
  data: VLref input; D output; Vin_fb input; Vout_fb input
function D = fcn(VLref,Vin_fb,Vout_fb)

D = min([1 max([0 (1 + (VLref - Vin_fb)/Vout_fb)])]);

== matlab function DCDC1_CL/VL2duty ==
  data: VLref input; D output; Vin_fb input; Vout_fb input
function D = fcn(VLref,Vin_fb,Vout_fb)

D = min([1 max([0 (1 + (VLref - Vin_fb)/Vout_fb)])]);

== matlab function DCDC1_CL/PWM with Dead Time1/MATLAB Function ==
  data: SH input; SHd input; SH output; SL output; SL input; SLd input
function [SH,SL] = fcn(SH,SHd,SL,SLd)

if SHd + SH > 1
    SH = 1;
else
    SH = 0;
end

if SLd + SL > 1
    SL = 1;
else
    SL = 0;
end

== matlab function DCDC1_CL/Iout2IL ==
  data: K_Iout_IL output; ILref input; IoutRef input; VoutRef input; Vin input; ILref output; RserL parameter
function [K_Iout_IL,ILref] = fcn(ILref,IoutRef,VoutRef,Vin,RserL)

if VoutRef < Vin
    VoutRef = Vin;
end
K_Iout_IL = (Vin - RserL*ILref) / VoutRef;
ILref = IoutRef / K_Iout_IL;

== matlab function DCDC1_CL/Iout2IL1 ==
  data: K_Iout_IL output; ILref input; IoutRef input; VoutRef input; Vin input; ILref output; RserL parameter
function [K_Iout_IL,ILref] = fcn(ILref,IoutRef,VoutRef,Vin,RserL)

if VoutRef < Vin
    VoutRef = Vin;
end
K_Iout_IL = (Vin - RserL*ILref) / VoutRef;
ILref = IoutRef / K_Iout_IL;

== matlab function DCDC1_CL/VL2duty1 ==
  data: VLref input; D output; Vin_fb input; Vout_fb input
function D = fcn(VLref,Vin_fb,Vout_fb)

D = min([1 max([0 (1 + (VLref - Vin_fb)/Vout_fb)])]);

== matlab function DCDC1_CL/Iout2IL2 ==
  data: K_Iout_IL output; ILref input; IoutRef input; VoutRef input; Vin input; ILref output; RserL parameter
function [K_Iout_IL,ILref] = fcn(ILref,IoutRef,VoutRef,Vin,RserL)

if VoutRef < Vin
    VoutRef = Vin;
end
K_Iout_IL = (Vin - RserL*ILref) / VoutRef;
ILref = IoutRef / K_Iout_IL;

== matlab function DCDC1_CL/Iout2IL3 ==
  data: K_Iout_IL output; ILref input; IoutRef input; VoutRef input; Vin input; ILref output; RserL parameter
function [K_Iout_IL,ILref] = fcn(ILref,IoutRef,VoutRef,Vin,RserL)

if VoutRef < Vin
    VoutRef = Vin;
end
K_Iout_IL = (Vin - RserL*ILref) / VoutRef;
ILref = IoutRef / K_Iout_IL;

== matlab function DCDC1_CL/VL2duty2 ==
  data: VLref input; D output; Vin_fb input; Vout_fb input; deadtimesw parameter; Tsw parameter
function D = fcn(VLref,Vin_fb,Vout_fb, deadtimesw, Tsw)

D = min([1 max([0 (1 + (VLref - Vin_fb)/Vout_fb + deadtimesw/Tsw)])]);
